simulink model "PracticeModel"  (R2013b)
settings: Solver=ode45  StartTime=0.0  StopTime=10.0  RelTol=1e-3
libraries: vrlib x1
settings Model: Creator=Deepak  LastModifiedBy=Deepak

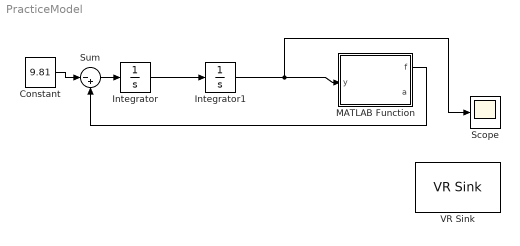
== system PracticeModel ==
  Constant : Constant  Value=9.81
  Integrator : Integrator
  Integrator1 : Integrator  InitialCondition=20
  MATLAB Function : MATLAB Function  TreatAsAtomicUnit=on
  Scope : Scope
      settings: TimeRange=10
  Sum : Sum  Inputs=|-+
  VR Sink : vrlib/VR Sink  InstantiateOnLoad=on  SampleTime=0.1  ViewEnable=on  RemoteChange=off  RemoteView=on  AutoView=off  VideoDimensions=[]  AllowVariableSize=off
  wires:
  Integrator/1 -> Integrator1/1
  Integrator1/1 -> Scope/1, MATLAB Function/1(y)
  Constant/1 -> Sum/1
  Sum/1 -> Integrator/1
  MATLAB Function/1(f) -> Sum/2

== matlab function PracticeModel/MATLAB Function ==
  data: y input; f output; a output
function [f,a] = fcn(y)
%#codegen
if y<1e-4
    y = 1e-4;
end
if y < 1.5
 f = 500*(1.5-y);
 a = sqrt(1.5^3/y);
else
    f = 0;
    a = 1.5;    
end
